simulink model "Chapter_1"  (R2021b)
settings: Solver=FixedStepDiscrete  StartTime=0.0  StopTime=1  FixedStep=0.01  RelTol=1e-3
settings Model: PacingRate=0.110000  Creator=win  LastModifiedBy=win

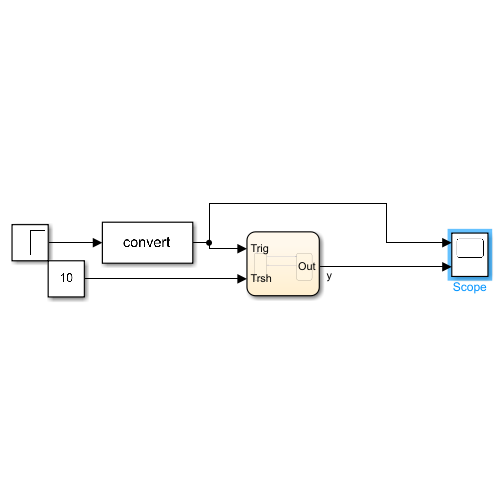
[thumbnail: Simulink's stored preview of the top-level diagram]
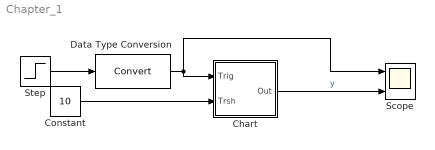
== system Chapter_1 ==
  Chart : Stateflow chart  TreatAsAtomicUnit=on
  Constant : Constant  Value=10
  Data Type Conversion : DataTypeConversion
  Scope : Scope  NumInputPorts=2
  Step : Step  Time=0.5  SampleTime=0
  wires:
  Chart/1(Out) -> Scope/2  "y"
  Step/1 -> Data Type Conversion/1
  Constant/1 -> Chart/2(Trsh)
  Data Type Conversion/1 -> Chart/1(Trig), Scope/1

== stateflow chart Chapter_1/Chart ==
  state Init
    during:
    Out=0;
  state Routine
    during:
    if cnt > Trsh
    Out =1;
    else
    cnt = cnt + 1;
    end
    exit:
    cnt =1;
  (default) -> Init
  Init -> Routine : [Trig == 1]{cnt =1;}
  Routine -> Init : [Trig == 0]
  data: Trig input; Out output; Trsh input; cnt local =1
